simulink model "Performance"  (R2024a)
settings: Solver=FixedStepAuto  StartTime=0.0  StopTime=12000  FixedStep=1  MaxStep=240.0  RelTol=1e-3
libraries: simulink x1
settings Model: Creator=Administrator  LastModifiedBy=kaguy
settings SolverCC: AlgebraicLoopSolver=TrustRegion
settings DebuggingCC: UnconnectedInputMsg=warning  UnconnectedOutputMsg=warning  UnconnectedLineMsg=warning
settings ModelReferenceCC: EnableRefExpFcnMdlSchedulingChecks=on
settings SFSimCC: CustomCodeUndefinedFunction=UseInterfaceOnly
settings RTWCC: GPUComputeCapability=3.5

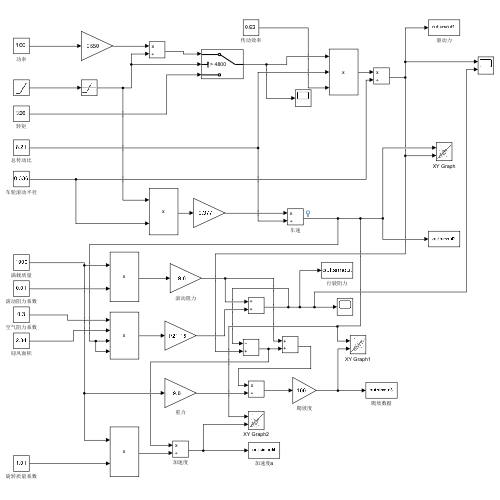
[thumbnail: Simulink's stored preview of the top-level diagram]
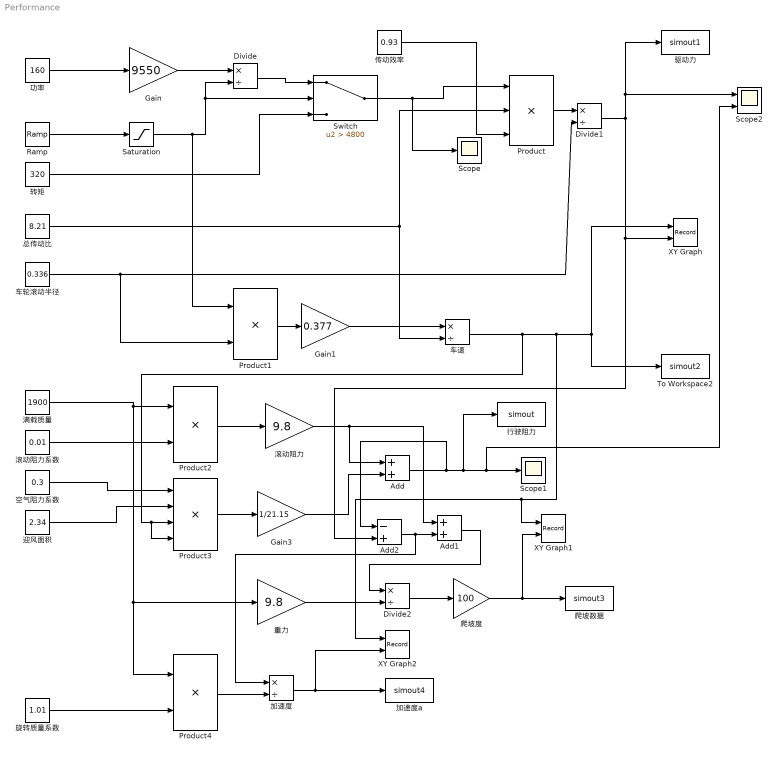
== system Performance ==
  Add : Sum
  Add1 : Sum
  Add2 : Sum  Inputs=-+
  Divide : Product  Inputs=*/
  Divide1 : Product  Inputs=*/
  Divide2 : Product  Inputs=*/
  Gain : Gain  Gain=9550
  Gain1 : Gain  Gain=0.377
  Gain3 : Gain  Gain=1/21.15
  Product : Product  Inputs=3
  Product1 : Product
  Product2 : Product
  Product3 : Product  Inputs=4
  Product4 : Product
  Ramp : simulink/Sources/Ramp  slope=1  start=0  InitialOutput=0
  Saturation : Saturate  UpperLimit=20000  LowerLimit=0
  Scope : Scope
  Scope1 : Scope
  Scope2 : Scope  NumInputPorts=2
  Switch : Switch  Criteria=u2 > Threshold  Threshold=4800  SaturateOnIntegerOverflow=off  InputSameDT=off
  To Workspace2 : ToWorkspace  VariableName=simout2  SaveFormat=Timeseries  SampleTime=-1
  XY Graph : Record  FileSettingsInternal="{\"entries\":[{\"content\":{\"excelSettings\":{\"content\":{},\"type\":\"Streamout.ExcelSettings\"}},\"type\":\"Streamout.FileSettingStorage\",\"uuid\":\"\"}],\"packageUris\":[\"http:\\/\\/schema.mathworks.com\\/mf0\\/streamout_blocks\\/R2020a\"],\"version\":\"1.0\"}"  Layout=[1 1]  SignalsInternal="{\"entries\":[{\"content\":{},\"type\":\"RecordBlkView.InputSignals\",\"uuid\":\"\"}],\"packageUris\":[\"http:\\/\\/schema.mathworks.com\\/mf0\\/streamout_blocks\\/R2020a\"],\"version\":\"1.0\"}"  VisualizationBindings="{\"xyplotplugin\":{\"info\":[{\"series\":[{\"bindingParametersList\":[{\"parameter\":\"X-Axis\",\"signalID\":2306,\"signalName\":\"车速\"},{\"parameter\":\"Y-Axis\",\"signalID\":2310,\"signalName\":\"Divide1\"}],\"seriesID\":0}],\"subplotID\":1}]}}"  CompatibilityTag=XY  st=-1
  XY Graph1 : Record  FileSettingsInternal="{\"entries\":[{\"content\":{\"excelSettings\":{\"content\":{},\"type\":\"Streamout.ExcelSettings\"}},\"type\":\"Streamout.FileSettingStorage\",\"uuid\":\"\"}],\"packageUris\":[\"http:\\/\\/schema.mathworks.com\\/mf0\\/streamout_blocks\\/R2020a\"],\"version\":\"1.0\"}"  Layout=[1 1]  SignalsInternal="{\"entries\":[{\"content\":{},\"type\":\"RecordBlkView.InputSignals\",\"uuid\":\"\"}],\"packageUris\":[\"http:\\/\\/schema.mathworks.com\\/mf0\\/streamout_blocks\\/R2020a\"],\"version\":\"1.0\"}"  VisualizationBindings="{\"xyplotplugin\":{\"info\":[{\"series\":[{\"bindingParametersList\":[{\"parameter\":\"X-Axis\",\"signalID\":2314,\"signalName\":\"车速\"},{\"parameter\":\"Y-Axis\",\"signalID\":2318,\"signalName\":\"爬坡度\"},{\"parameter\":\"X-Axis\",\"signalID\":2314,\"signalName\":\"车速\"},{\"parameter\":\"Y-Axis\",\"signalID\":2318,\"signalName\":\"爬坡度\"}],\"seriesID\":0}],\"subplotID\":1}]}}"  CompatibilityTag=XY  st=-1
  XY Graph2 : Record  FileSettingsInternal="{\"entries\":[{\"content\":{\"excelSettings\":{\"content\":{},\"type\":\"Streamout.ExcelSettings\"}},\"type\":\"Streamout.FileSettingStorage\",\"uuid\":\"\"}],\"packageUris\":[\"http:\\/\\/schema.mathworks.com\\/mf0\\/streamout_blocks\\/R2020a\"],\"version\":\"1.0\"}"  Layout=[1 1]  SignalsInternal="{\"entries\":[{\"content\":{\"signals\":[{\"content\":{\"blockPath\":[],\"dimensions\":[1],\"domain\":\"\",\"lineColor\":\"#000000\",\"port\":1,\"sid\":[\"\"],\"signalID\":1,\"signalName\":\"车速\"},\"type\":\"RecordBlkView.Signal\",\"uuid\":\"\"},{\"content\":{\"blockPath\":[],\"dimensions\":[1],\"domain\":\"\",\"lineColor\":\"#000000\",\"port\":2,\"sid\":[\"\"],\"signalID\":2,\"signalName\":\"Divide1\"},\"type\":\"RecordBlkView.Signal\",\"uuid\":\"\"},{\"content\":{\"blockPath\":[],\"dimensions\":[1],\"domain\":\"\",\"lineColor\":\"#000000\",\"port\":1,\"sid\":[\"\"],\"signalID\":3,\"signalName\":\"车速\"},\"type\":\"RecordBlkView.Signal\",\"uuid\":\"\"},{\"content\":{\"blockPath\":[],\"dimensions\":[1],\"domain\":\"\",\"lineColor\":\"#000000\",\"port\":2,\"sid\":[\"\"],\"signalID\":4,\"signalName\":\"爬坡度\"},\"type\":\"RecordBlkView.Signal\",\"uuid\":\"\"},{\"content\":{\"blockPath\":[],\"dimensions\":[1],\"domain\":\"\",\"lineColor\":\"#000000\",\"plots\":[ 1 ],\"port\":1,\"sid\":[\"\"],\"signalID\":5,\"signalName\":\"车速\"},\"type\":\"RecordBlkView.Signal\",\"uuid\":\"\"},{\"content\":{\"blockPath\":[],\"dimensions\":[1],\"domain\":\"\",\"lineColor\":\"#000000\",\"plots\":[ 1 ],\"port\":2,\"sid\":[\"\"],\"signalID\":6,\"signalName\":\"加速度\"},\"type\":\"RecordBlkView.Signal\",\"uuid\":\"\"},{\"content\":{\"blockPath\":[],\"dimensions\":[1],\"domain\":\"\",\"lineColor\":\"#000000\",\"lineWidth\":2,\"port\":1,\"sid\":[\"\"],\"signalID\":7,\"signalName\":\"车速\"},\"type\":\"RecordBlkView.Signal\",\"uuid\":\"\"},{\"content\":{\"blockPath\":[],\"dimensions\":[1],\"domain\":\"\",\"lineColor\":\"#000000\",\"lineWidth\":2,\"port\":1,\"sid\":[\"\"],\"signalID\":8,\"signalName\":\"加速度\"},\"type\":\"RecordBlkView.Signal\",\"uuid\":\"\"},{\"content\":{\"blockPath\":[],\"dimensions\":[1],\"domain\":\"\",\"lineColor\":\"#b746ff\",\"lineWidth\":2,\"port\":1,\"sid\":[\"\"],\"signalID\":9,\"signalName\":\"爬坡度\"},\"type\":\"RecordBlkView.Signal\",\"uuid\":\"\"},{\"content\":{\"blockPath\":[],\"dimensions\":[1],\"domain\":\"\",\"lineColor\":\"#000000\",\"lineStyle\":\"DASH_DOT\",\"port\":1,\"sid\":[\"\"],\"signalID\":10,\"signalName\":\"Add\"},\"type\":\"RecordBlkView.Signal\",\"uuid\":\"\"},{\"content\":{\"blockPath\":[],\"dimensions\":[1],\"domain\":\"\",\"lineColor\":\"#000000\",\"port\":1,\"sid\":[\"\"],\"signalID\":11,\"signalName\":\"Divide1\"},\"type\":\"RecordBlkView.Signal\",\"uuid\":\"\"}]},\"type\":\"RecordBlkView.InputSignals\",\"uuid\":\"\"}],\"packageUris\":[\"http:\\/\\/schema.mathworks.com\\/mf0\\/streamout_blocks\\/R2020a\"],\"version\":\"1.0\"}"  VisualizationBindings="{\"xyplotplugin\":{\"info\":[{\"series\":[{\"bindingParametersList\":[{\"parameter\":\"X-Axis\",\"signalID\":5,\"signalName\":\"车速\"},{\"parameter\":\"Y-Axis\",\"signalID\":6,\"signalName\":\"加速度\"}],\"seriesID\":0}],\"subplotID\":1}]}}"  CompatibilityTag=XY  st=-1
  传动效率 : Constant  Value=0.93
  功率 : Constant  Value=160
  加速度 : Product  Inputs=*/
  加速度a : ToWorkspace  VariableName=simout4  SaveFormat=Timeseries  SampleTime=-1
  总传动比 : Constant  Value=8.21
  旋转质量系数 : Constant  Value=1.01
  滚动阻力 : Gain  Gain=9.8
  滚动阻力系数 : Constant  Value=0.01
  满载质量 : Constant  Value=1900
  爬坡度 : Gain  Gain=100
  爬坡数据 : ToWorkspace  VariableName=simout3  SaveFormat=Timeseries  SampleTime=-1
  空气阻力系数 : Constant  Value=0.3
  行驶阻力 : ToWorkspace  VariableName=simout  SaveFormat=Timeseries  SampleTime=-1
  车轮滚动半径 : Constant  Value=0.336
  车速 : Product  Inputs=*/
  转矩 : Constant  Value=320
  迎风面积 : Constant  Value=2.34
  重力 : Gain  Gain=9.8
  驱动力 : ToWorkspace  VariableName=simout1  SaveFormat=Timeseries  SampleTime=-1
  wires:
  Gain/1 -> Divide/1
  功率/1 -> Gain/1
  Ramp/1 -> Saturation/1
  Saturation/1 -> Product1/1, Divide/2, Switch/2
  Divide/1 -> Switch/1
  转矩/1 -> Switch/3
  Switch/1 -> Scope/1, Product/1
  总传动比/1 -> 车速/2, Product/2
  传动效率/1 -> Product/3
  Product/1 -> Divide1/1
  车轮滚动半径/1 -> Product1/2, Divide1/2
  Product1/1 -> Gain1/1
  Gain1/1 -> 车速/1
  车速/1 -> Product3/4, Product3/3, XY Graph2/1, XY Graph1/1, To Workspace2/1, XY Graph/1
  Divide1/1 -> 驱动力/1, Scope2/1, Add2/2, XY Graph/2
  满载质量/1 -> Product4/1, 重力/1, Product2/1
  滚动阻力系数/1 -> Product2/2
  Product2/1 -> 滚动阻力/1
  空气阻力系数/1 -> Product3/1
  迎风面积/1 -> Product3/2
  Product3/1 -> Gain3/1
  滚动阻力/1 -> Add1/1, Add/1
  Gain3/1 -> Add/2
  Add/1 -> Add2/1, 行驶阻力/1, Scope2/2, Scope1/1
  重力/1 -> Divide2/2
  Divide2/1 -> 爬坡度/1
  爬坡度/1 -> XY Graph1/2, 爬坡数据/1
  Add2/1 -> 加速度/1, Add1/2
  Add1/1 -> Divide2/1
  旋转质量系数/1 -> Product4/2
  Product4/1 -> 加速度/2
  加速度/1 -> XY Graph2/2, 加速度a/1
